simulink model "position_controller_62"  (R2021a)
settings: Solver=VariableStepAuto  StartTime=0.0  StopTime=10.0  RelTol=1e-3
values from neighbouring files (symbols this model uses):
  g = sqrt((obj.position(1)-obj.parent.position(1))^2 +                       (obj.position(2)-obj.parent.position(2))^2 +                       (obj.position(3)-obj.parent.position(3))^2)    [node.m]
undefined symbols (not defined in the file or in its folder): k_e, k_x, mass_total
settings Model: Creator=Marcus  LastModifiedBy=Marcus

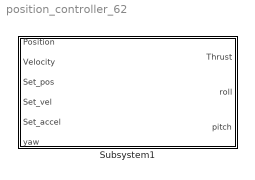
== system position_controller_62 ==
  Subsystem1 : Subsystem

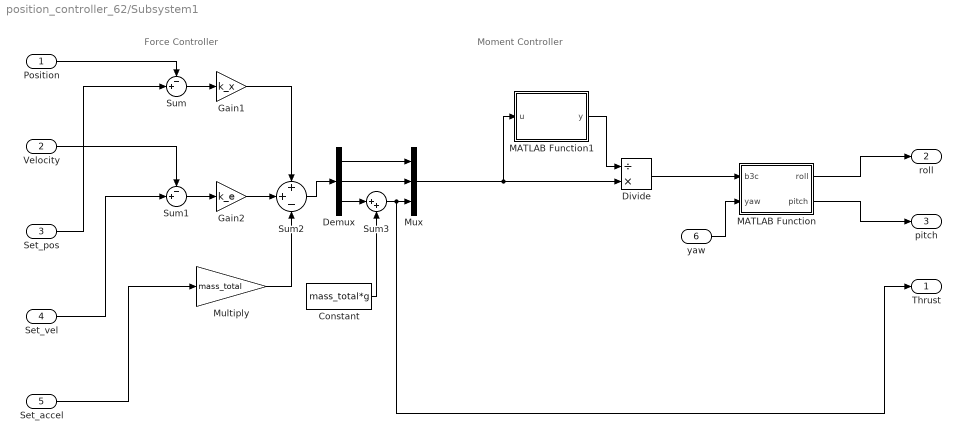
== system position_controller_62/Subsystem1 ==
  note: Moment Controller
  note: Force Controller
  Position : Inport
  Velocity : Inport  Port=2
  Set_pos : Inport  Port=3
  Set_vel : Inport  Port=4
  Set_accel : Inport  Port=5
  yaw : Inport  Port=6
  Constant : Constant  Value=mass_total*g
  Demux : Demux  Outputs=3
  Divide : Product  Inputs=/*
  Gain1 : Gain  Gain=k_x
  Gain2 : Gain  Gain=k_e
  MATLAB Function : MATLAB Function  TreatAsAtomicUnit=on
  MATLAB Function1 : MATLAB Function  TreatAsAtomicUnit=on
  Multiply : Gain  Gain=mass_total
  Mux : Mux  Inputs=3
  Sum : Sum  Inputs=-+|
  Sum1 : Sum  Inputs=-+|
  Sum2 : Sum  Inputs=++-
  Sum3 : Sum  Inputs=|++
  Thrust : Outport
  roll : Outport  Port=2
  pitch : Outport  Port=3
  wires:
  Sum/1 -> Gain1/1
  Position/1 -> Sum/1
  Set_pos/1 -> Sum/2
  Sum1/1 -> Gain2/1
  Velocity/1 -> Sum1/1
  Set_vel/1 -> Sum1/2
  Gain1/1 -> Sum2/1
  Gain2/1 -> Sum2/2
  Set_accel/1 -> Multiply/1
  Multiply/1 -> Sum2/3
  Sum2/1 -> Demux/1
  Demux/1 -> Mux/1
  Demux/2 -> Mux/2
  Sum3/1 -> Thrust/1, Mux/3
  Demux/3 -> Sum3/1
  Constant/1 -> Sum3/2
  Mux/1 -> MATLAB Function1/1(u), Divide/2
  MATLAB Function1/1(y) -> Divide/1
  Divide/1 -> MATLAB Function/1(b3c)
  yaw/1 -> MATLAB Function/2(yaw)
  MATLAB Function/1(roll) -> roll/1
  MATLAB Function/2(pitch) -> pitch/1

== matlab function position_controller_62/Subsystem1/MATLAB Function ==
  data: b3c input; roll output; yaw input; pitch output
function [roll, pitch] = calc(b3c, yaw)

yaw_dt = yaw + pi/2;

b3a = cross([cos(yaw_dt); sin(yaw_dt); 0], b3c);
b3b = cross(b3c, b3a);

angles = rotm2eul([b3a b3b b3c], 'ZYX');

roll = angles(3); pitch = angles(2);

== matlab function position_controller_62/Subsystem1/MATLAB Function1 ==
  data: u input; y output
function y = norm(u)
y = norm(u);
